simulink model "DecimationChainSSR"  (R2023a)
settings: Solver=VariableStepAuto  StartTime=0.0  StopTime=5000  RelTol=1e-3
undefined symbols (not defined in the file): Asymmetric, cfi, hb1, hb2, hb3, S, Shift1, Shift2, Shift3, ShiftCF, vsva2197, xcvc1902
libraries: aieBasic x10, aieDSP x4, dspmlti4 x3, dspsrcs4 x1, aieUtilities x1, vmcUtilities x1
settings Model: Creator=robg  LastModifiedBy=robg
settings DebuggingCC: UnconnectedInputMsg=warning  UnconnectedOutputMsg=warning  UnconnectedLineMsg=warning
settings ModelReferenceCC: EnableRefExpFcnMdlSchedulingChecks=on
settings RTWCC: DLArmComputeVersion=19.05

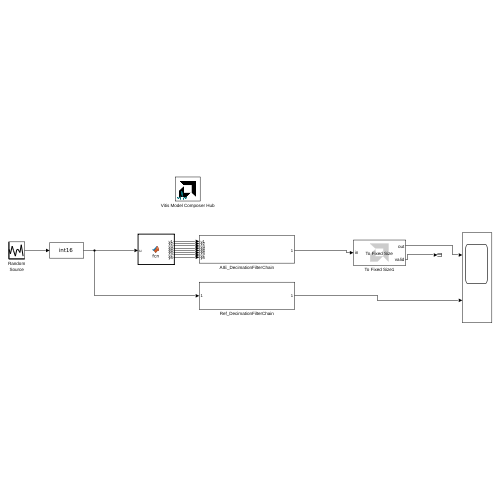
[thumbnail: Simulink's stored preview of the top-level diagram]
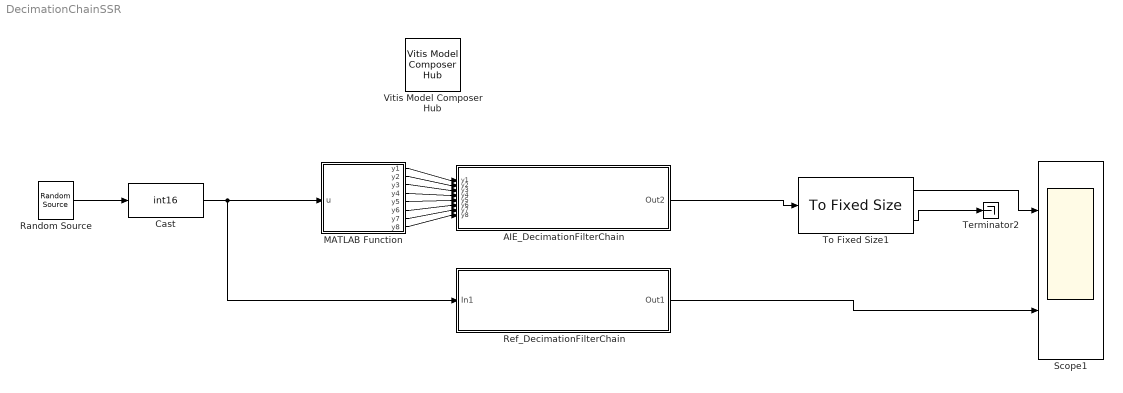
== system DecimationChainSSR ==
  AIE_DecimationFilterChain : Subsystem
  Cast : DataTypeConversion  OutDataTypeStr=int16  SaturateOnIntegerOverflow=off  RndMeth=Floor
  MATLAB Function : MATLAB Function  TreatAsAtomicUnit=on
  Random Source : dspsrcs4/Random Source  SrcType=Uniform  NormMethod=Ziggurat  CltLength=12  MinVal=-3e4  MaxVal=3e4  MeanVal=0  VarVal=1  RepMode=Not repeatable  rawSeed=1  IsInherit=off  SampMode=Discrete  SampTime=1  SampFrame=2048  DataType=Double  OutComplex=Complex  OutputFrames=off
  Ref_DecimationFilterChain : Subsystem
  Scope1 : Scope  NumInputPorts=2
  Terminator2 : Terminator
  To Fixed Size1 : aieUtilities/To Fixed Size  Mode=Produce a valid output signal  OutputSize=Inherit: Same as input  CopyMethod=Buffer samples to form output  HasStatusOutput=on
  Vitis Model Composer Hub : vmcUtilities/Vitis Model Composer Hub  Tag=genX  CodeGeneration=off  SubsystemName=FIRchain_stream  StartColumn=1  NumberOfColumns=1  TargetDirectory=./code_stream  exportDesign=off  analyzeDesign=off  validateDesignOnHw=off  ExportType=AI Engines  IpVendor=xilinx.com  IpLibrary=hls  IpVersion=1.0  IpHWLanguage=Verilog  AieCompilerOptions={'--Xmapper=disableFloorplanning', '--verbose'}  AieSimulatorOptions={}  CreateTestbench=on  TestbenchStackSize=10  RunRtlSim=off  RunCSim=off  RunAieSim=on  AieSimTimeout=10000  RunAieSimProfiling=on  LaunchVitisAnalyzer=on  PlotOutput=on  RunX86Sim=off  X86SimTimeout=10  GenHwImage=off  GenLibadfXo=off  GenHwValidationCode=off  PlatformType=Specify Platform  Platform=/proj/xbuilds/SWIP/9999.0_0118_1552/installs/lin64/Vitis/2023.1/base_platforms/xilinx_vck190_base_202310_1/xilinx_vck190_base_202310_1.xpfm  HwSystemType=Baremetal  HwValidationTarget=hw  ProjDevice=Versal VCK190 Evaluation Platform (xcvc1902-vsva2197-2MP-e-S)  ProjDevicePart=xcvc1902-vsva2197-2MP-e-S  AIEType=AIE  SamplePeriod=-1  ClockFrequency=200  DataPathParallelism=1  xilinxfamily=versalaicore  part=xcvc1902  speed=-2MP-e-S  package=vsva2197  directory=./netlist  testbench=off  incr_netlist=off  synthesis_tool=Vivado  clock_wrapper=Clock Enables  dbl_ovrd=According to Block Masks  dcm_input_clock_period=10  sysclk_period=10  simulink_period=1  eval_field=0  LogFileName=''  NThreads=4
  wires:
  Random Source/1 -> Cast/1
  Cast/1 -> Ref_DecimationFilterChain/1(In1), MATLAB Function/1(u)
  MATLAB Function/1(y1) -> AIE_DecimationFilterChain/1(y1)
  MATLAB Function/2(y2) -> AIE_DecimationFilterChain/2(y2)
  AIE_DecimationFilterChain/1(Out2) -> To Fixed Size1/1
  To Fixed Size1/2 -> Terminator2/1
  MATLAB Function/3(y3) -> AIE_DecimationFilterChain/3(y3)
  MATLAB Function/4(y4) -> AIE_DecimationFilterChain/4(y4)
  MATLAB Function/5(y5) -> AIE_DecimationFilterChain/5(y5)
  MATLAB Function/6(y6) -> AIE_DecimationFilterChain/6(y6)
  MATLAB Function/7(y7) -> AIE_DecimationFilterChain/7(y7)
  MATLAB Function/8(y8) -> AIE_DecimationFilterChain/8(y8)
  To Fixed Size1/1 -> Scope1/1
  Ref_DecimationFilterChain/1(Out1) -> Scope1/2

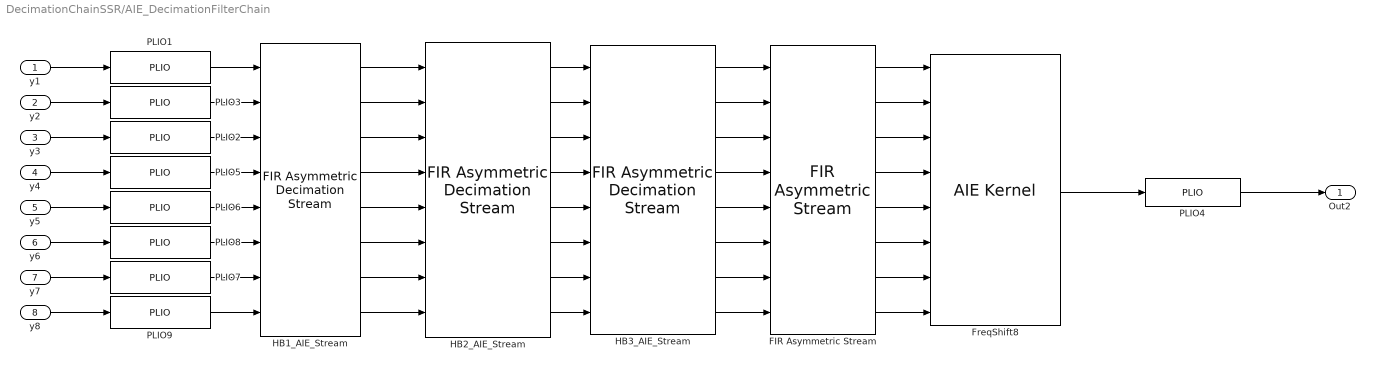
== system DecimationChainSSR/AIE_DecimationFilterChain ==
  y1 : Inport
  y2 : Inport  Port=2
  y3 : Inport  Port=3
  y4 : Inport  Port=4
  y5 : Inport  Port=5
  y6 : Inport  Port=6
  y7 : Inport  Port=7
  y8 : Inport  Port=8
  FIR Asymmetric Stream : aieDSP/FIR Asymmetric Stream  data_type=cint16  coef_type=int16  use_coeff_reload=off  dual_ip=off  num_outputs=off  coeff=cfi  fir_length=28  input_window_size=256  shift_val=ShiftCF  rnd_mode=Round to positive infinity  sat_mode=1-Asymmetric  ssr=8  casc_length=1  AIE_VARIANT=1  blockJsonConstraints=[]  blockJsonConstraintsInternal=[]  spec=vmc_stream_fir_sr_asym.json  SerializedMaskParamNames=[]  SerializedMaskParamValues=[]  SerializedMaskParamVisibilities=[]  block_type=FIR Asymmetric Stream  SerializedMaskParamDataypes=typename|typename|bool|bool|bool|coef_type|uint|uint|uint|uint|uint|uint|uint|uint  SerializedMaskParamEnumStrArr=0|0|0|0|0|0|0|0|0|Floor,Ceiling,Round to positive infinity,Round to negative infinity,Round symmetrical to infinity,Round symmetrical to zero,Round convergent to even,Round convergent to odd|0-None,1-Asymmetric,3-Symmetric|0|0|0  SerializedMaskParamEnumValArr=0|0|0|0|0|0|0|0|0|0,1,2,3,4,5,6,7|0,1,3|0|0|0  SerializedMaskParamVectorArr=0|0|0|0|0|1|0|0|0|0|0|0|0|0
  FreqShift8 : aieBasic/AIE Kernel  KernelAllAttrs=|  PortNames={'in1'; 'in2'; 'in3'; 'in4'; 'in5'; 'in6'; 'in7'; 'in8'; 'out'}  PortSerializedTypes={'{Q2{R{Tadf::input_buffer{1{t{Scint16}}}}}}'; '{Q2{R{Tadf::input_buffer{1{t{Scint16}}}}}}'; '{Q2{R{Tadf::input_buffer{1{t{Scint16}}}}}}'; '{Q2{R{Tadf::input_buffer{1{t{Scint16}}}}}}'; '{Q2{R{Tadf::input_buffer{1{t{Scint16}}}}}}'; '{Q2{R{Tadf::input_buffer{1{t{Scint16}}}}}}'; '{Q2{R{Tadf::input_buffer{1{t{Scint16}}}}}}'; '{Q2{R{Tadf::input_buffer{1{t{Scint16}}}}}}'; '{Q2{R{Tadf::output_buffer{1{t{Scint16}}}}}}'}  PortWindowSizes={3.200000000000000000e+01, 3.200000000000000000e+01, 3.200000000000000000e+01, 3.200000000000000000e+01, 3.200000000000000000e+01, 3.200000000000000000e+01, 3.200000000000000000e+01, 3.200000000000000000e+01, 2.560000000000000000e+02}  PortWindowMargins={0.000000000000000000e+00, 0.000000000000000000e+00, 0.000000000000000000e+00, 0.000000000000000000e+00, 0.000000000000000000e+00, 0.000000000000000000e+00, 0.000000000000000000e+00, 0.000000000000000000e+00, 0.000000000000000000e+00}  PortSynchronicities={'sync', 'sync', 'sync', 'sync', 'sync', 'sync', 'sync', 'sync', 'sync'}  PortSignalSizes={0.000000000000000000e+00; 0.000000000000000000e+00; 0.000000000000000000e+00; 0.000000000000000000e+00; 0.000000000000000000e+00; 0.000000000000000000e+00; 0.000000000000000000e+00; 0.000000000000000000e+00; 0.000000000000000000e+00}  FunctionTemplateSpecKind=implicit  FunctionTemplateParamNames={'FRAME_LENGTH'}  FunctionTemplateParamKinds={'nontype'}  FunctionTemplateParamTypes={'int'}  FunctionTemplateParamValues={'256'}  FunctionIndex=1  FunctionTabVisible=on  FunctionTemplateParamsVisible=on  FunctionDeclTypeOptions=|  FunctionDecl=|  FunctionTemplateParams={ 'FRAME_LENGTH', 'int', '256' }  FunctionTemplateParamsEnables={'off', 'off', 'on'}  PortAttrs={ 'input', 'in1', 'adf::input_buffer< cint16 > & restrict', '32', '0', 'sync', ''; 'input', 'in2', 'adf::input_buffer< cint16 > & restrict', '32', '0', 'sync', ''; 'input', 'in3', 'adf::input_buffer< cint16 > & restrict', '32', '0', 'sync', ''; 'input', 'in4', 'adf::input_buffer< cint16 > & restrict', '32', '0', 'sync', ''; 'input', 'in5', 'adf::input_buffer< cint16 > & restrict', '32', '0', 'sync', ''; 'input', 'in6', 'adf::input_buffer< cint16 > & restrict', '32', '0', 'sync', ''; 'input', 'in7', 'adf::input_buffer< cint16 > & restrict', '32', '0', 'sync', ''; 'input', 'in8', 'adf::input_buffer< cint16 > & restrict', '32', '0', 'sync', ''; 'output', 'out', 'adf::output_buffer< cint16 > & restrict', '256', '', 'sync', '' }  PortAttrsEnables={'off', 'off', 'off', 'on', 'off', 'off', 'off';'off', 'off', 'off', 'on', 'off', 'off', 'off';'off', 'off', 'off', 'on', 'off', 'off', 'off';'off', 'off', 'off', 'on', 'off', 'off', 'off';'off', 'off', 'off', 'on', 'off', 'off', 'off';'off', 'off', 'off', 'on', 'off', 'off', 'off';'off', 'off', 'off', 'on', 'off', 'off', 'off';'off', 'off', 'off', 'on', 'off', 'off', 'off';'off', 'off', 'off', 'on', 'off', 'off', 'off'}  SampleTime=-1  KernelHeaderFile=FreqShift.h  KernelFunction=FreqShift8  KernelSourceFile=FreqShift.cpp  KernelSearchPaths={'$AIESRC'}  PreProcOptions={}  blockJsonConstraints=[]
      KernelAllAttrs=|
      | s[12;12;9;9;19;14;21;23;21;23;24;21;15;17;12;24;26;26;26;27;28;9;21;23;23;23;24;25;14;19;19;29]@FunctionNameDeclFileNamePortNamesPortTypesPortSerializedTypesPortDirectionsPortWindowSizeEnablesPortWindowMarginEnablesPortBufferSizeEnablesPortBufferMarginEnablesPortSynchronicityEnablesPortSignalSizeEnablesPortBufferSizesPortBufferMarginsFunctionDeclFunctionTemplateSpecKindFunctionTemplateParamNamesFunctionTemplateParamKindsFunctionTemplateParamTypesFunctionTemplateParamValuesFunctionTemplateParamEnablesClassDeclClassTemplateSpecKindClassTemplateParamNamesClassTemplateParamKindsClassTemplateParamTypesClassTemplateParamValuesClassTemplateParamEnablesClassCtorDeclsClassCtorParamNamesClassCtorParamTypesClassCtorParamSerializedTypes[1 1]@C[32 1]@t10@FreqShift8t113@/proj/xcoswmktg/robg/git/AIEngine_Library/01-Introduction_to_Versal_ACAP_and_AI_Engines/../common/src/FreqShift.hC[9 1]@t3@in1t3@in2t3@in3t3@in4t3@in5t3@in6t3@in7t3@in8t3@outC[9 1]@t38@adf::input_buffer< cint16 > & restrictt38@adf::input_buffer< cint16 > & restrictt38@adf::input_buffer< cint16 > & restrictt38@adf::input_buffer< cint16 > & restrictt38@adf::input_buffer< cint16 > & restrictt38@adf::input_buffer< cint16 > & restrictt38@adf::input_buffer< cint16 > & restrictt38@adf::input_buffer< cint16 > & restrictt39@adf::output_buffer< cint16 > & restrictC[9 1]@t42@{Q2{R{Tadf::input_buffer{1{t{Scint16}}}}}}t42@{Q2{R{Tadf::input_buffer{1{t{Scint16}}}}}}t42@{Q2{R{Tadf::input_buffer{1{t{Scint16}}}}}}t42@{Q2{R{Tadf::input_buffer{1{t{Scint16}}}}}}t42@{Q2{R{Tadf::input_buffer{1{t{Scint16}}}}}}t42@{Q2{R{Tadf::input_buffer{1{t{Scint16}}}}}}t42@{Q2{R{Tadf::input_buffer{1{t{Scint16}}}}}}t42@{Q2{R{Tadf::input_buffer{1{t{Scint16}}}}}}t43@{Q2{R{Tadf::output_buffer{1{t{Scint16}}}}}}C[9 1]@t5@inputt5@inputt5@inputt5@inputt5@inputt5@inputt5@inputt5@inputt6@outputC[9 1]@l1@l1@l1@l1@l1@l1@l1@l1@l1@C[9 1]@l1@l1@l1@l1@l1@l1@l1@l1@l0@C[9 1]@l1@l1@l1@l1@l1@l1@l1@l1@l1@C[9 1]@l0@l0@l0@l0@l0@l0@l0@l0@l0@C[9 1]@l1@l1@l1@l1@l1@l1@l1@l1@l1@C[9 1]@l0@l0@l0@l0@l0@l0@l0@l0@l0@C[9 1]@nnnnnnnnnC[9 1]@nnnnnnnnnt443@template < int FRAME_LENGTH > 
      | void FreqShift8(adf::input_buffer< cint16 > & restrict in1, adf::input_buffer< cint16 > & restrict in2, adf::input_buffer< cint16 > & restrict in3, adf::input_buffer< cint16 > & restrict in4, adf::input_buffer< cint16 > & restrict in5, adf::input_buffer< cint16 > & restrict in6, adf::input_buffer< cint16 > & restrict in7, adf::input_buffer< cint16 > & restrict in8, adf::output_buffer< cint16 > & restrict out)t8@implicitC[1 1]@t12@FRAME_LENGTHC[1 1]@t7@nontypeC[1 1]@t3@intC[1 1]@nC[1 1]@l1@nne[0 1]@e[0 1]@e[0 1]@e[0 1]@e[0 1]@e[0 1]@e[0 1]@e[0 1]@e[0 1]@
      FunctionDeclTypeOptions=|
      | C[1 1]@t452@template < int FRAME_LENGTH > 
      | void FreqShift8(adf::input_buffer< cint16 > && restrict in1, adf::input_buffer< cint16 > && restrict in2, adf::input_buffer< cint16 > && restrict in3, adf::input_buffer< cint16 > && restrict in4, adf::input_buffer< cint16 > && restrict in5, adf::input_buffer< cint16 > && restrict in6, adf::input_buffer< cint16 > && restrict in7, adf::input_buffer< cint16 > && restrict in8, adf::output_buffer< cint16 > && restrict out)
      FunctionDecl=|
      | template < int FRAME_LENGTH > 
      | void FreqShift8(adf::input_buffer< cint16 > && restrict in1, adf::input_buffer< cint16 > && restrict in2, adf::input_buffer< cint16 > && restrict in3, adf::input_buffer< cint16 > && restrict in4, adf::input_buffer< cint16 > && restrict in5, adf::input_buffer< cint16 > && restrict in6, adf::input_buffer< cint16 > && restrict in7, adf::input_buffer< cint16 > && restrict in8, adf::output_buffer< cint16 > && restrict out)
  HB1_AIE_Stream : aieDSP/FIR Asymmetric Decimation Stream  data_type=cint16  coef_type=int16  use_coeff_reload=off  dual_ip=off  num_outputs=off  coeff=hb1  fir_length=26  decimate_factor=2  input_window_size=2048  shift_val=Shift1  rnd_mode=Floor  sat_mode=1-Asymmetric  ssr=8  deci_poly=1  casc_length=1  AIE_VARIANT=1  blockJsonConstraints="{\"type\":\"constraint\",\"constraintType\":\"location_graph\",\"sid\":\"59\",\"lhs\":{\"type\":\"location\",\"templParam\":\"graph\",\"args\":{\"type\":\"kernel\",\"name\":\"ChannelizerStream/FIRchain_stream/HB1_AIE_Stream\",\"sid\":\"59\"}},\"rhs\":{\"type\":\"grouparea\",\"args\":{\"type\":\"group\",\"groups\":{\"type\":\"array\",\"args\":{\"type\":\"group\",\"tiletype\":\"aie\",\"colmin\":{\"type\":\"evaluable\",\"expr\":\"6\",\"value\":6},\"rowmin\":{\"type\":\"evaluable\",\"expr\":\"0\",\"value\":0},\"colmax\":{\"type\":\"evaluable\",\"expr\":\"13\",\"value\":13},\"rowmax\":{\"type\":\"evaluable\",\"expr\":\"7\",\"value\":7}}},\"containrouting\":false,\"exclusiverouting\":false,\"exclusiveplacement\":false}},\"equality\":true}"  blockJsonConstraintsInternal=[]  spec=vmc_stream_fir_decimate_asym.json  SerializedMaskParamNames=[]  SerializedMaskParamValues=[]  SerializedMaskParamVisibilities=[]  block_type=FIR Asymmetric Decimation Stream  SerializedMaskParamDataypes=typename|typename|bool|bool|bool|coef_type|uint|uint|uint|uint|uint|uint|uint|uint|uint|uint  SerializedMaskParamEnumStrArr=0|0|0|0|0|0|0|0|0|0|Floor,Ceiling,Round to positive infinity,Round to negative infinity,Round symmetrical to infinity,Round symmetrical to zero,Round convergent to even,Round convergent to odd|0-None,1-Asymmetric,3-Symmetric|0|0|0|0  SerializedMaskParamEnumValArr=0|0|0|0|0|0|0|0|0|0|0,1,2,3,4,5,6,7|0,1,3|0|0|0|0  SerializedMaskParamVectorArr=0|0|0|0|0|1|0|0|0|0|0|0|0|0|0|0
  HB2_AIE_Stream : aieDSP/FIR Asymmetric Decimation Stream  data_type=cint16  coef_type=int16  use_coeff_reload=off  dual_ip=off  num_outputs=off  coeff=hb2  fir_length=26  decimate_factor=2  input_window_size=1024  shift_val=Shift2  rnd_mode=Floor  sat_mode=1-Asymmetric  ssr=8  deci_poly=1  casc_length=1  AIE_VARIANT=1  blockJsonConstraints="{\"type\":\"constraint\",\"constraintType\":\"location_graph\",\"sid\":\"60\",\"lhs\":{\"type\":\"location\",\"templParam\":\"graph\",\"args\":{\"type\":\"kernel\",\"name\":\"ChannelizerStream/FIRchain_stream/HB2_AIE_Stream\",\"sid\":\"60\"}},\"rhs\":{\"type\":\"grouparea\",\"args\":{\"type\":\"group\",\"groups\":{\"type\":\"array\",\"args\":{\"type\":\"group\",\"tiletype\":\"aie\",\"colmin\":{\"type\":\"evaluable\",\"expr\":\"14\",\"value\":14},\"rowmin\":{\"type\":\"evaluable\",\"expr\":\"0\",\"value\":0},\"colmax\":{\"type\":\"evaluable\",\"expr\":\"21\",\"value\":21},\"rowmax\":{\"type\":\"evaluable\",\"expr\":\"7\",\"value\":7}}},\"containrouting\":false,\"exclusiverouting\":false,\"exclusiveplacement\":false}},\"equality\":true}"  blockJsonConstraintsInternal=[]  spec=vmc_stream_fir_decimate_asym.json  SerializedMaskParamNames=[]  SerializedMaskParamValues=[]  SerializedMaskParamVisibilities=[]  block_type=FIR Asymmetric Decimation Stream  SerializedMaskParamDataypes=typename|typename|bool|bool|bool|coef_type|uint|uint|uint|uint|uint|uint|uint|uint|uint|uint  SerializedMaskParamEnumStrArr=0|0|0|0|0|0|0|0|0|0|Floor,Ceiling,Round to positive infinity,Round to negative infinity,Round symmetrical to infinity,Round symmetrical to zero,Round convergent to even,Round convergent to odd|0-None,1-Asymmetric,3-Symmetric|0|0|0|0  SerializedMaskParamEnumValArr=0|0|0|0|0|0|0|0|0|0|0,1,2,3,4,5,6,7|0,1,3|0|0|0|0  SerializedMaskParamVectorArr=0|0|0|0|0|1|0|0|0|0|0|0|0|0|0|0
  HB3_AIE_Stream : aieDSP/FIR Asymmetric Decimation Stream  data_type=cint16  coef_type=int16  use_coeff_reload=off  dual_ip=off  num_outputs=off  coeff=hb3  fir_length=26  decimate_factor=2  input_window_size=512  shift_val=Shift3  rnd_mode=Floor  sat_mode=1-Asymmetric  ssr=8  deci_poly=1  casc_length=1  AIE_VARIANT=1  blockJsonConstraints="{\"type\":\"constraint\",\"constraintType\":\"location_graph\",\"sid\":\"61\",\"lhs\":{\"type\":\"location\",\"templParam\":\"graph\",\"args\":{\"type\":\"kernel\",\"name\":\"ChannelizerStream/FIRchain_stream/HB3_AIE_Stream\",\"sid\":\"61\"}},\"rhs\":{\"type\":\"grouparea\",\"args\":{\"type\":\"group\",\"groups\":{\"type\":\"array\",\"args\":{\"type\":\"group\",\"tiletype\":\"aie\",\"colmin\":{\"type\":\"evaluable\",\"expr\":\"22\",\"value\":22},\"rowmin\":{\"type\":\"evaluable\",\"expr\":\"0\",\"value\":0},\"colmax\":{\"type\":\"evaluable\",\"expr\":\"29\",\"value\":29},\"rowmax\":{\"type\":\"evaluable\",\"expr\":\"7\",\"value\":7}}},\"containrouting\":false,\"exclusiverouting\":false,\"exclusiveplacement\":false}},\"equality\":true}"  blockJsonConstraintsInternal=[]  spec=vmc_stream_fir_decimate_asym.json  SerializedMaskParamNames=[]  SerializedMaskParamValues=[]  SerializedMaskParamVisibilities=[]  block_type=FIR Asymmetric Decimation Stream  SerializedMaskParamDataypes=typename|typename|bool|bool|bool|coef_type|uint|uint|uint|uint|uint|uint|uint|uint|uint|uint  SerializedMaskParamEnumStrArr=0|0|0|0|0|0|0|0|0|0|Floor,Ceiling,Round to positive infinity,Round to negative infinity,Round symmetrical to infinity,Round symmetrical to zero,Round convergent to even,Round convergent to odd|0-None,1-Asymmetric,3-Symmetric|0|0|0|0  SerializedMaskParamEnumValArr=0|0|0|0|0|0|0|0|0|0|0,1,2,3,4,5,6,7|0,1,3|0|0|0|0  SerializedMaskParamVectorArr=0|0|0|0|0|1|0|0|0|0|0|0|0|0|0|0
  PLIO{1..9} (9 alike) : aieBasic/PLIO  PlioWidth=128  PlioFreqSpec=on  PlioFreq=250  ColLocation=0  channel=0  blockJsonConstraints=[]  deprecateConstraints=0
  Out2 : Outport
  wires:
  PLIO3/1 -> HB1_AIE_Stream/2
  HB3_AIE_Stream/1 -> FIR Asymmetric Stream/1
  HB2_AIE_Stream/2 -> HB3_AIE_Stream/2
  HB3_AIE_Stream/2 -> FIR Asymmetric Stream/2
  HB1_AIE_Stream/2 -> HB2_AIE_Stream/2
  y1/1 -> PLIO1/1
  HB2_AIE_Stream/1 -> HB3_AIE_Stream/1
  PLIO1/1 -> HB1_AIE_Stream/1
  PLIO4/1 -> Out2/1
  y2/1 -> PLIO3/1
  FreqShift8/1 -> PLIO4/1
  HB1_AIE_Stream/1 -> HB2_AIE_Stream/1
  FIR Asymmetric Stream/1 -> FreqShift8/1
  FIR Asymmetric Stream/2 -> FreqShift8/2
  y4/1 -> PLIO5/1
  y3/1 -> PLIO2/1
  y7/1 -> PLIO7/1
  y8/1 -> PLIO9/1
  y6/1 -> PLIO8/1
  y5/1 -> PLIO6/1
  PLIO2/1 -> HB1_AIE_Stream/3
  PLIO5/1 -> HB1_AIE_Stream/4
  PLIO6/1 -> HB1_AIE_Stream/5
  PLIO7/1 -> HB1_AIE_Stream/7
  PLIO9/1 -> HB1_AIE_Stream/8
  HB1_AIE_Stream/3 -> HB2_AIE_Stream/3
  HB1_AIE_Stream/4 -> HB2_AIE_Stream/4
  HB1_AIE_Stream/5 -> HB2_AIE_Stream/5
  HB1_AIE_Stream/6 -> HB2_AIE_Stream/6
  HB1_AIE_Stream/7 -> HB2_AIE_Stream/7
  HB1_AIE_Stream/8 -> HB2_AIE_Stream/8
  HB2_AIE_Stream/3 -> HB3_AIE_Stream/3
  HB2_AIE_Stream/4 -> HB3_AIE_Stream/4
  HB2_AIE_Stream/5 -> HB3_AIE_Stream/5
  HB2_AIE_Stream/6 -> HB3_AIE_Stream/6
  HB2_AIE_Stream/7 -> HB3_AIE_Stream/7
  HB2_AIE_Stream/8 -> HB3_AIE_Stream/8
  HB3_AIE_Stream/3 -> FIR Asymmetric Stream/3
  HB3_AIE_Stream/4 -> FIR Asymmetric Stream/4
  HB3_AIE_Stream/5 -> FIR Asymmetric Stream/5
  HB3_AIE_Stream/6 -> FIR Asymmetric Stream/6
  HB3_AIE_Stream/7 -> FIR Asymmetric Stream/7
  HB3_AIE_Stream/8 -> FIR Asymmetric Stream/8
  PLIO8/1 -> HB1_AIE_Stream/6
  FIR Asymmetric Stream/3 -> FreqShift8/3
  FIR Asymmetric Stream/4 -> FreqShift8/4
  FIR Asymmetric Stream/5 -> FreqShift8/5
  FIR Asymmetric Stream/6 -> FreqShift8/6
  FIR Asymmetric Stream/7 -> FreqShift8/7
  FIR Asymmetric Stream/8 -> FreqShift8/8

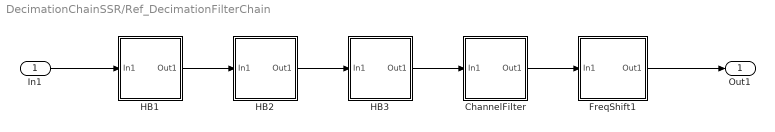
== system DecimationChainSSR/Ref_DecimationFilterChain ==
  In1 : Inport
  ChannelFilter : Subsystem  mask{COEFFS=cfi, Shift=ShiftCF}
      mask prompts: COEFFS "Coefficients"; Shift "Final Shift"
  FreqShift1 : Subsystem
  HB1 : Subsystem  mask{COEFFS=hb1, Shift=Shift1}
      mask prompts: COEFFS "Coefficients"; Shift "Final Shift"
  HB2 : Subsystem  mask{COEFFS=hb2, Shift=Shift2}
      mask prompts: COEFFS "Coefficients"; Shift "Final Shift"
  HB3 : Subsystem  mask{COEFFS=hb3, Shift=Shift3}
      mask prompts: COEFFS "Coefficients"; Shift "Final Shift"
  Out1 : Outport
  wires:
  ChannelFilter/1(Out1) -> FreqShift1/1(In1)
  HB1/1(Out1) -> HB2/1(In1)
  HB2/1(Out1) -> HB3/1(In1)
  FreqShift1/1(Out1) -> Out1/1
  HB3/1(Out1) -> ChannelFilter/1(In1)
  In1/1 -> HB1/1(In1)

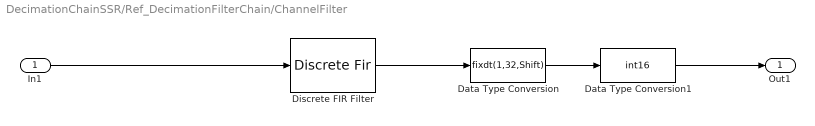
== system DecimationChainSSR/Ref_DecimationFilterChain/ChannelFilter ==
  In1 : Inport
  Data Type Conversion : DataTypeConversion  OutDataTypeStr=fixdt(1,32,Shift)  ConvertRealWorld=Stored Integer (SI)  SaturateOnIntegerOverflow=off  RndMeth=Floor
  Data Type Conversion1 : DataTypeConversion  OutDataTypeStr=int16  RndMeth=Floor
  Discrete FIR Filter : DiscreteFir  Coefficients=COEFFS  InputProcessing=Columns as channels (frame based)
  Out1 : Outport
  wires:
  Data Type Conversion1/1 -> Out1/1
  Discrete FIR Filter/1 -> Data Type Conversion/1
  In1/1 -> Discrete FIR Filter/1
  Data Type Conversion/1 -> Data Type Conversion1/1

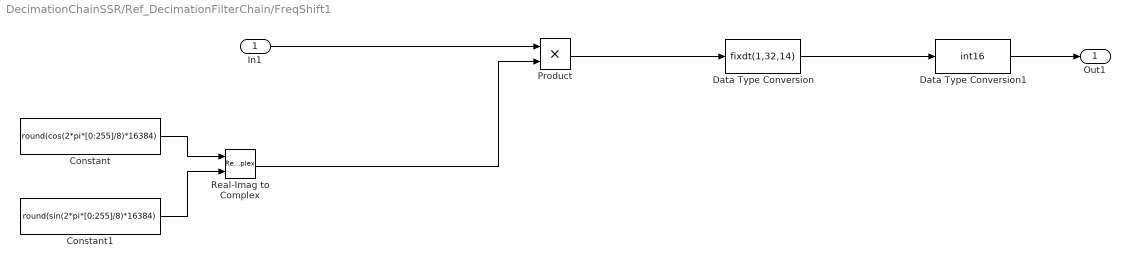
== system DecimationChainSSR/Ref_DecimationFilterChain/FreqShift1 ==
  In1 : Inport
  Constant : Constant  Value=round(cos(2*pi*[0:255]/8)*16384)  SampleTime=2048
  Constant1 : Constant  Value=round(sin(2*pi*[0:255]/8)*16384)  SampleTime=2048
  Data Type Conversion : DataTypeConversion  OutDataTypeStr=fixdt(1,32,14)  ConvertRealWorld=Stored Integer (SI)  SaturateOnIntegerOverflow=off  RndMeth=Floor
  Data Type Conversion1 : DataTypeConversion  OutDataTypeStr=int16  RndMeth=Floor
  Product : Product
  Real-Imag to Complex : RealImagToComplex
  Out1 : Outport
  wires:
  Data Type Conversion/1 -> Data Type Conversion1/1
  Constant1/1 -> Real-Imag to Complex/2
  Constant/1 -> Real-Imag to Complex/1
  Data Type Conversion1/1 -> Out1/1
  Real-Imag to Complex/1 -> Product/2
  Product/1 -> Data Type Conversion/1
  In1/1 -> Product/1

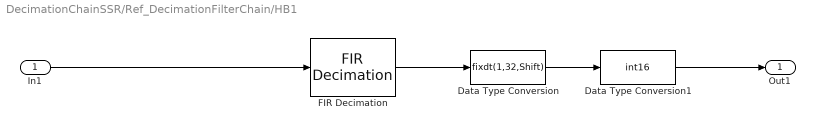
== system DecimationChainSSR/Ref_DecimationFilterChain/HB1 ==
  In1 : Inport
  Data Type Conversion : DataTypeConversion  OutDataTypeStr=fixdt(1,32,Shift)  ConvertRealWorld=Stored Integer (SI)  SaturateOnIntegerOverflow=off  RndMeth=Floor
  Data Type Conversion1 : DataTypeConversion  OutDataTypeStr=int16  RndMeth=Floor
  FIR Decimation : dspmlti4/FIR Decimation  FilterSource=Dialog parameters  h=COEFFS  D=2  filtStruct=Direct form  FilterObject=FDECIM  InputProcessing=Columns as channels (frame based)  framing=Enforce single-rate processing  AllowArbitraryInputLength=off  inputOffset=0  outputBufInitCond=0  roundingMode=Floor  overflowMode=off  firstCoeffDataTypeStr=Inherit: Same word length as input  firstCoeffMin=[]  firstCoeffMax=[]  firstCoeffLastDataTypeStr=Inherit: Same word length as input  outputDataTypeStr=Inherit: Same as accumulator  outputMin=[]  outputMax=[]  outputLastDataTypeStr=Inherit: Same as accumulator
  Out1 : Outport
  wires:
  Data Type Conversion1/1 -> Out1/1
  FIR Decimation/1 -> Data Type Conversion/1
  In1/1 -> FIR Decimation/1
  Data Type Conversion/1 -> Data Type Conversion1/1

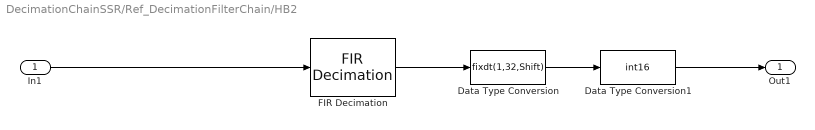
== system DecimationChainSSR/Ref_DecimationFilterChain/HB2 ==
  In1 : Inport
  Data Type Conversion : DataTypeConversion  OutDataTypeStr=fixdt(1,32,Shift)  ConvertRealWorld=Stored Integer (SI)  SaturateOnIntegerOverflow=off  RndMeth=Floor
  Data Type Conversion1 : DataTypeConversion  OutDataTypeStr=int16  RndMeth=Floor
  FIR Decimation : dspmlti4/FIR Decimation  FilterSource=Dialog parameters  h=COEFFS  D=2  filtStruct=Direct form  FilterObject=FDECIM  InputProcessing=Columns as channels (frame based)  framing=Enforce single-rate processing  AllowArbitraryInputLength=off  inputOffset=0  outputBufInitCond=0  roundingMode=Floor  overflowMode=off  firstCoeffDataTypeStr=Inherit: Same word length as input  firstCoeffMin=[]  firstCoeffMax=[]  firstCoeffLastDataTypeStr=Inherit: Same word length as input  outputDataTypeStr=Inherit: Same as accumulator  outputMin=[]  outputMax=[]  outputLastDataTypeStr=Inherit: Same as accumulator
  Out1 : Outport
  wires:
  Data Type Conversion1/1 -> Out1/1
  FIR Decimation/1 -> Data Type Conversion/1
  In1/1 -> FIR Decimation/1
  Data Type Conversion/1 -> Data Type Conversion1/1

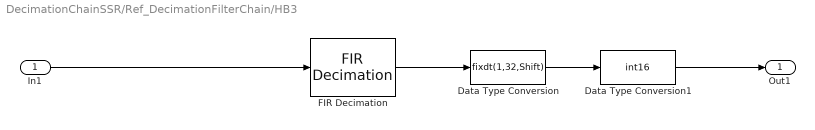
== system DecimationChainSSR/Ref_DecimationFilterChain/HB3 ==
  In1 : Inport
  Data Type Conversion : DataTypeConversion  OutDataTypeStr=fixdt(1,32,Shift)  ConvertRealWorld=Stored Integer (SI)  SaturateOnIntegerOverflow=off  RndMeth=Floor
  Data Type Conversion1 : DataTypeConversion  OutDataTypeStr=int16  RndMeth=Floor
  FIR Decimation : dspmlti4/FIR Decimation  FilterSource=Dialog parameters  h=COEFFS  D=2  filtStruct=Direct form  FilterObject=FDECIM  InputProcessing=Columns as channels (frame based)  framing=Enforce single-rate processing  AllowArbitraryInputLength=off  inputOffset=0  outputBufInitCond=0  roundingMode=Floor  overflowMode=off  firstCoeffDataTypeStr=Inherit: Same word length as input  firstCoeffMin=[]  firstCoeffMax=[]  firstCoeffLastDataTypeStr=Inherit: Same word length as input  outputDataTypeStr=Inherit: Same as accumulator  outputMin=[]  outputMax=[]  outputLastDataTypeStr=Inherit: Same as accumulator
  Out1 : Outport
  wires:
  Data Type Conversion/1 -> Data Type Conversion1/1
  In1/1 -> FIR Decimation/1
  FIR Decimation/1 -> Data Type Conversion/1
  Data Type Conversion1/1 -> Out1/1

== matlab function DecimationChainSSR/MATLAB Function ==
  data: u input; y1 output; y2 output; y3 output; y4 output; y5 output; y6 output; y7 output; y8 output
function [y1,y2,y3,y4,y5,y6,y7,y8] = fcn(u)

y1 = u(1:8:end);
y2 = u(2:8:end);
y3 = u(3:8:end);
y4 = u(4:8:end);
y5 = u(5:8:end);
y6 = u(6:8:end);
y7 = u(7:8:end);
y8 = u(8:8:end);
